simulink model "model"  (R2025b)
settings: Solver=VariableStepAuto  StartTime=0.0  StopTime=10.0  RelTol=1e-3
values from neighbouring files (symbols this model uses):
  A_inv = 1 / A    (= 0.25)    [script.m]
  den = [Tv 1]    [script.m]
  k_valve = S * sqrt(2 * g)    [script.m]
  num = 1    [script.m]
  Qin = 10 / 1000    (= 0.01)    [script.m]
  Qin_step = 10    [script.m]
  T_step = 25000    [script.m]
  z1_0 = 0.5    [script.m]
  z2_0 = 0.5    [script.m]
settings Model: Creator=Vladimir  LastModifiedBy=Vladimir

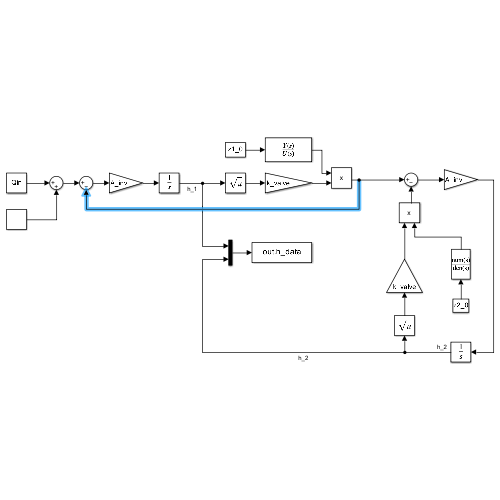
[thumbnail: Simulink's stored preview of the top-level diagram]
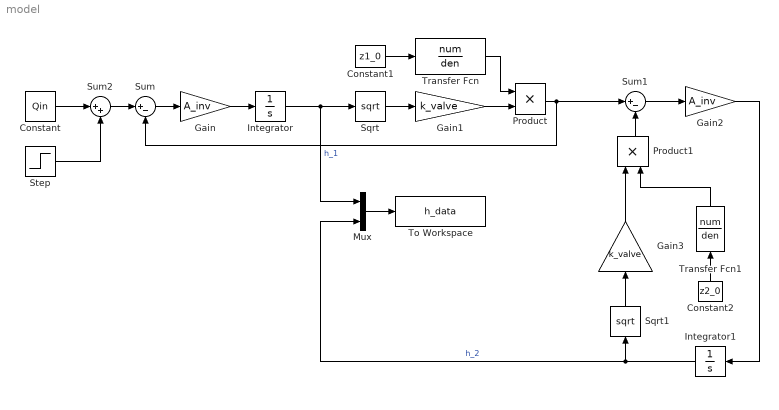
== system model ==
  Constant : Constant  Value=Qin
  Constant1 : Constant  Value=z1_0
  Constant2 : Constant  Value=z2_0
  Gain : Gain  Gain=A_inv
  Gain1 : Gain  Gain=k_valve
  Gain2 : Gain  Gain=A_inv
  Gain3 : Gain  Gain=k_valve
  Integrator : Integrator
  Integrator1 : Integrator
  Mux : Mux  Inputs=2
  Product : Product
  Product1 : Product
  Sqrt : Sqrt
  Sqrt1 : Sqrt
  Step : Step  Time=T_step  After=Qin_step / 10000  SampleTime=0
  Sum : Sum  Inputs=|+-
  Sum1 : Sum  Inputs=|+-
  Sum2 : Sum  Inputs=|++
  To Workspace : ToWorkspace  VariableName=h_data  SaveFormat=Timeseries  SampleTime=-1
  Transfer Fcn : TransferFcn  Numerator=num  Denominator=den
  Transfer Fcn1 : TransferFcn  Numerator=num  Denominator=den
  wires:
  Constant/1 -> Sum2/1
  Sum/1 -> Gain/1
  Gain/1 -> Integrator/1
  Integrator/1 -> Sqrt/1, Mux/1  "h_1"
  Sqrt/1 -> Gain1/1
  Sum1/1 -> Gain2/1
  Gain2/1 -> Integrator1/1
  Integrator1/1 -> Mux/2, Sqrt1/1  "h_2"
  Sqrt1/1 -> Gain3/1
  Mux/1 -> To Workspace/1
  Gain1/1 -> Product/2
  Product/1 -> Sum1/1, Sum/2
  Product1/1 -> Sum1/2
  Constant2/1 -> Transfer Fcn1/1
  Gain3/1 -> Product1/1
  Step/1 -> Sum2/2
  Sum2/1 -> Sum/1
  Constant1/1 -> Transfer Fcn/1
  Transfer Fcn/1 -> Product/1
  Transfer Fcn1/1 -> Product1/2
